simulink model "gm_HDL_pfc_gold_fi"  (R2024b)
settings: Solver=FixedStepDiscrete  StartTime=0.0  StopTime=.06  RelTol=1e-3
InitFcn:
  | fidelity_pfc_vals;
  | load('C:\Users\angro\Desktop\hil\pfc3ph\matlab\sim\sschdl\pfc_desktop\stateSpaceParameters.mat');
undefined symbols (not defined in the file or in its folder): a, b, c, fsw, t_ss, tsw
libraries: simulink x38, hdlmdlgenlib x26, hdlsllib x9, mcbcontrolslib x5, dspsrcs4 x3, slpidlib x2, spsSVPWMGenerator2LevelLib x1, spsPLL3phLib x1
(part 1 of 4)
settings Model: Creator=angro  LastModifiedBy=angro
settings OptimizationCC: BlockReduction=off  ConditionallyExecuteInputs=off  DefaultParameterBehavior=Inlined  InheritOutputTypeSmallerThanSingle=on
settings DebuggingCC: SignalRangeChecking=warning  AlgebraicLoopMsg=error  ArtificialAlgebraicLoopMsg=error  InheritedTsInSrcMsg=none  SingleTaskRateTransMsg=error  UnconnectedInputMsg=warning  UnconnectedOutputMsg=warning  UnconnectedLineMsg=warning
settings HardwareCC: ProdBitPerPointer=32  ProdBitPerSizeT=32  ProdBitPerPtrDiffT=32  ProdLargestAtomicFloat=None  ProdIntDivRoundTo=Undefined  ProdEndianess=Unspecified  ProdWordSize=32  ProdHWDeviceType=ASIC/FPGA->ASIC/FPGA  TargetBitPerPointer=64  TargetBitPerSizeT=64  TargetBitPerPtrDiffT=64  TargetLongLongMode=on  TargetIntDivRoundTo=Zero  TargetEndianess=LittleEndian  TargetWordSize=64  TargetHWDeviceType=Custom Processor->MATLAB Host Computer  ProdEqTarget=off

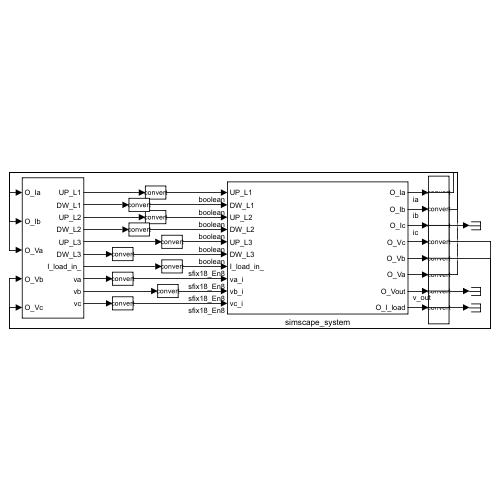
[thumbnail: Simulink's stored preview of the top-level diagram]
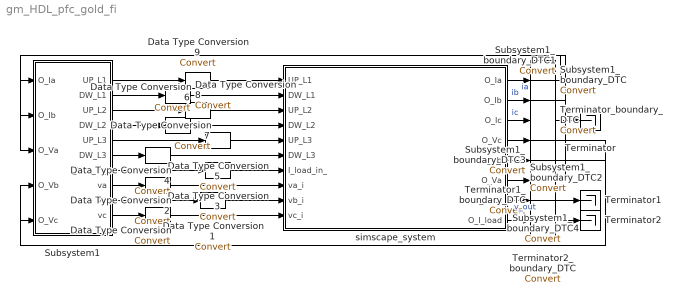
== system gm_HDL_pfc_gold_fi ==
  Data Type Conversion{,1..9} (10 alike) : DataTypeConversion  SaturateOnIntegerOverflow=off  RndMeth=Floor
  Subsystem1 : Subsystem
  Subsystem1_boundary_DTC{,1..4} (5 alike) : DataTypeConversion
  Terminator : Terminator
  Terminator1 : Terminator
  Terminator1_boundary_DTC : DataTypeConversion
  Terminator2 : Terminator
  Terminator2_boundary_DTC : DataTypeConversion
  Terminator_boundary_DTC : DataTypeConversion
  simscape_system : Subsystem
  wires:
  Terminator2_boundary_DTC/1 -> Terminator2/1
  simscape_system/8(O_I_load) -> Terminator2_boundary_DTC/1
  Terminator1_boundary_DTC/1 -> Terminator1/1
  simscape_system/7(O_Vout) -> Terminator1_boundary_DTC/1  "v_out"
  Subsystem1_boundary_DTC4/1 -> Subsystem1/3(O_Va)
  simscape_system/6(O_Va) -> Subsystem1_boundary_DTC4/1
  Subsystem1_boundary_DTC3/1 -> Subsystem1/4(O_Vb)
  simscape_system/5(O_Vb) -> Subsystem1_boundary_DTC3/1
  Subsystem1_boundary_DTC2/1 -> Subsystem1/5(O_Vc)
  simscape_system/4(O_Vc) -> Subsystem1_boundary_DTC2/1
  Terminator_boundary_DTC/1 -> Terminator/1
  simscape_system/3(O_Ic) -> Terminator_boundary_DTC/1  "ic"
  Subsystem1_boundary_DTC1/1 -> Subsystem1/2(O_Ib)
  simscape_system/2(O_Ib) -> Subsystem1_boundary_DTC1/1  "ib"
  Subsystem1_boundary_DTC/1 -> Subsystem1/1(O_Ia)
  simscape_system/1(O_Ia) -> Subsystem1_boundary_DTC/1  "ia"
  Data Type Conversion9/1 -> simscape_system/1(UP_L1)
  Data Type Conversion8/1 -> simscape_system/2(DW_L1)
  Data Type Conversion7/1 -> simscape_system/3(UP_L2)
  Data Type Conversion6/1 -> simscape_system/4(DW_L2)
  Data Type Conversion5/1 -> simscape_system/5(UP_L3)
  Data Type Conversion4/1 -> simscape_system/6(DW_L3)
  Data Type Conversion3/1 -> simscape_system/7(I_load_in_)
  Data Type Conversion2/1 -> simscape_system/8(va_i)
  Data Type Conversion1/1 -> simscape_system/9(vb_i)
  Data Type Conversion/1 -> simscape_system/10(vc_i)
  Subsystem1/10(vc) -> Data Type Conversion/1
  Subsystem1/9(vb) -> Data Type Conversion1/1
  Subsystem1/8(va) -> Data Type Conversion2/1
  Subsystem1/6(DW_L3) -> Data Type Conversion4/1
  Subsystem1/5(UP_L3) -> Data Type Conversion5/1
  Subsystem1/4(DW_L2) -> Data Type Conversion6/1
  Subsystem1/3(UP_L2) -> Data Type Conversion7/1
  Subsystem1/2(DW_L1) -> Data Type Conversion8/1
  Subsystem1/1(UP_L1) -> Data Type Conversion9/1
  Subsystem1/7(I_load_in_) -> Data Type Conversion3/1

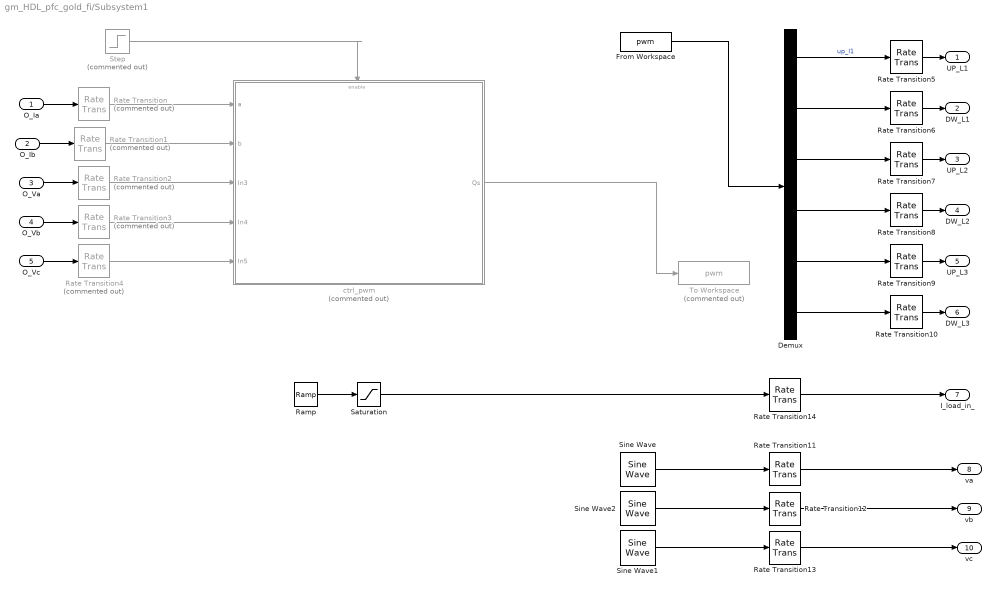
== system gm_HDL_pfc_gold_fi/Subsystem1 ==
  O_Ia : Inport
  O_Ib : Inport  Port=2
  O_Va : Inport  Port=3
  O_Vb : Inport  Port=4
  O_Vc : Inport  Port=5
  Demux : Demux  Outputs=6
  From Workspace : FromWorkspace  VariableName=pwm  SampleTime=t_ss  Interpolate=off  ZeroCross=off  OutputAfterFinalValue=Holding final value
  Ramp : simulink/Sources/Ramp  slope=1/50  start=2/50  InitialOutput=0
  Rate Transition{,1..4} (5 alike) : RateTransition  Commented=on  OutPortSampleTime=t_ss
  Rate Transition{5..10,14} (7 alike) : RateTransition  OutPortSampleTime=t_ss
  Rate Transition11 : RateTransition
  Rate Transition12 : RateTransition
  Rate Transition13 : RateTransition
  Saturation : Saturate  UpperLimit=2
  Sine Wave : dspsrcs4/Sine Wave  Amplitude=325  Frequency=50  Phase=0  SampleMode=Discrete  OutComplex=Real  CompMethod=Table lookup  TableSize=Speed  SampleTime=tsw  SamplesPerFrame=1  ResetState=Restart at time zero  OutputFrames=off  dataType=double  wordLen=16  udDataType=sfix(16)  fracBitsMode=Best precision  numFracBits=15  OutDataTypeStr=double  LastOutDataTypeStr=double
  Sine Wave1 : dspsrcs4/Sine Wave  Amplitude=325  Frequency=50  Phase=2*pi/3  SampleMode=Discrete  OutComplex=Real  CompMethod=Table lookup  TableSize=Speed  SampleTime=tsw  SamplesPerFrame=1  ResetState=Restart at time zero  OutputFrames=off  dataType=double  wordLen=16  udDataType=sfix(16)  fracBitsMode=Best precision  numFracBits=15  OutDataTypeStr=double  LastOutDataTypeStr=double
  Sine Wave2 : dspsrcs4/Sine Wave  Amplitude=325  Frequency=50  Phase=-2*pi/3  SampleMode=Discrete  OutComplex=Real  CompMethod=Table lookup  TableSize=Speed  SampleTime=tsw  SamplesPerFrame=1  ResetState=Restart at time zero  OutputFrames=off  dataType=double  wordLen=16  udDataType=sfix(16)  fracBitsMode=Best precision  numFracBits=15  OutDataTypeStr=double  LastOutDataTypeStr=double
  Step : Step  Commented=on  Time=2/50  SampleTime=0
  To Workspace : ToWorkspace  Commented=on  VariableName=pwm  SaveFormat=Timeseries  SampleTime=-1
  ctrl_pwm : Subsystem  Commented=on
  UP_L1 : Outport
  DW_L1 : Outport  Port=2
  UP_L2 : Outport  Port=3
  DW_L2 : Outport  Port=4
  UP_L3 : Outport  Port=5
  DW_L3 : Outport  Port=6
  I_load_in_ : Outport  Port=7
  va : Outport  Port=8
  vb : Outport  Port=9
  vc : Outport  Port=10
  wires:
  From Workspace/1 -> Demux/1
  Ramp/1 -> Saturation/1
  Rate Transition14/1 -> I_load_in_/1
  Step/1 -> ctrl_pwm/Enable
  Rate Transition4/1 -> ctrl_pwm/5(In5)
  Rate Transition3/1 -> ctrl_pwm/4(In4)
  Rate Transition2/1 -> ctrl_pwm/3(In3)
  Rate Transition1/1 -> ctrl_pwm/2(b)
  Rate Transition/1 -> ctrl_pwm/1(a)
  ctrl_pwm/1(Qs) -> To Workspace/1
  Rate Transition13/1 -> vc/1
  Rate Transition12/1 -> vb/1
  Rate Transition11/1 -> va/1
  Sine Wave1/1 -> Rate Transition13/1
  Sine Wave2/1 -> Rate Transition12/1
  Sine Wave/1 -> Rate Transition11/1
  Saturation/1 -> Rate Transition14/1
  Rate Transition10/1 -> DW_L3/1
  Rate Transition9/1 -> UP_L3/1
  Rate Transition8/1 -> DW_L2/1
  Rate Transition7/1 -> UP_L2/1
  Rate Transition6/1 -> DW_L1/1
  Rate Transition5/1 -> UP_L1/1
  O_Vc/1 -> Rate Transition4/1
  O_Vb/1 -> Rate Transition3/1
  O_Va/1 -> Rate Transition2/1
  O_Ib/1 -> Rate Transition1/1
  O_Ia/1 -> Rate Transition/1
  Demux/2 -> Rate Transition6/1
  Demux/3 -> Rate Transition7/1
  Demux/4 -> Rate Transition8/1
  Demux/6 -> Rate Transition10/1
  Demux/1 -> Rate Transition5/1  "up_l1"
  Demux/5 -> Rate Transition9/1

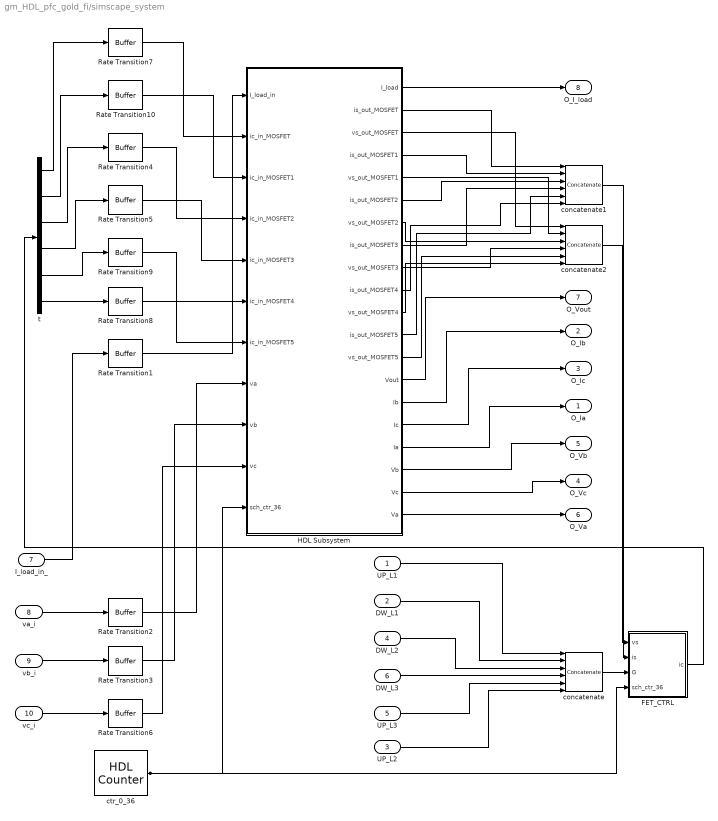
== system gm_HDL_pfc_gold_fi/simscape_system ==
  UP_L1 : Inport  OutDataTypeStr=boolean  PortDimensions=1  SampleTime=5.12820512820513e-07
  DW_L1 : Inport  Port=2  OutDataTypeStr=boolean  PortDimensions=1  SampleTime=5.12820512820513e-07
  UP_L2 : Inport  Port=3  OutDataTypeStr=boolean  PortDimensions=1  SampleTime=5.12820512820513e-07
  DW_L2 : Inport  Port=4  OutDataTypeStr=boolean  PortDimensions=1  SampleTime=5.12820512820513e-07
  UP_L3 : Inport  Port=5  OutDataTypeStr=boolean  PortDimensions=1  SampleTime=5.12820512820513e-07
  DW_L3 : Inport  Port=6  OutDataTypeStr=boolean  PortDimensions=1  SampleTime=5.12820512820513e-07
  I_load_in_ : Inport  Port=7  OutDataTypeStr=fixdt(1, 18, 8)  PortDimensions=1  SampleTime=5.12820512820513e-07
  va_i : Inport  Port=8  OutDataTypeStr=fixdt(1, 18, 8)  PortDimensions=1  SampleTime=5.12820512820513e-07  LockScale=on
  vb_i : Inport  Port=9  OutDataTypeStr=fixdt(1, 18, 8)  PortDimensions=1  SampleTime=5.12820512820513e-07  LockScale=on
  vc_i : Inport  Port=10  OutDataTypeStr=fixdt(1, 18, 8)  PortDimensions=1  SampleTime=5.12820512820513e-07  LockScale=on
  FET_CTRL : Subsystem
  HDL Subsystem : Subsystem
  Rate Transition{1..10} (10 alike) : hdlmdlgenlib/Buffer
  concatenate : Concatenate  NumInputs=6
  concatenate1 : Concatenate  NumInputs=6
  concatenate2 : Concatenate  NumInputs=6
  ctr_0_36 : hdlsllib/Sources/HDL Counter  CountType=Count limited  CountInit=double(0)  CountStep=double(1)  CountMax=double(36)  CountFromType=Initial value  CountFrom=double(0)  CountResetPort=off  CountLoadPort=off  CountEnbPort=off  CountDirPort=off  CountHitOutputPort=off  CountDataType=Unsigned  CountWordLen=6  CountFracLen=0  CountSampTime=1.38600138600139e-08
  t : Demux  Outputs=6
  O_Ia : Outport  SampleTime=5.12820512820513e-07
  O_Ib : Outport  Port=2  SampleTime=5.12820512820513e-07
  O_Ic : Outport  Port=3  SampleTime=5.12820512820513e-07
  O_Vc : Outport  Port=4  SampleTime=5.12820512820513e-07
  O_Vb : Outport  Port=5  SampleTime=5.12820512820513e-07
  O_Va : Outport  Port=6  SampleTime=5.12820512820513e-07
  O_Vout : Outport  Port=7  SampleTime=5.12820512820513e-07
  O_I_load : Outport  Port=8  SampleTime=5.12820512820513e-07
  wires:
  t/1 -> Rate Transition7/1
  t/2 -> Rate Transition10/1
  va_i/1 -> Rate Transition2/1
  concatenate/1 -> FET_CTRL/3(G)
  HDL Subsystem/12(is_out_MOSFET5) -> concatenate1/5
  t/3 -> Rate Transition4/1
  t/4 -> Rate Transition5/1
  t/5 -> Rate Transition9/1
  t/6 -> Rate Transition8/1
  I_load_in_/1 -> Rate Transition1/1
  UP_L1/1 -> concatenate/1
  vb_i/1 -> Rate Transition3/1
  DW_L1/1 -> concatenate/2
  Rate Transition2/1 -> HDL Subsystem/8(va)
  vc_i/1 -> Rate Transition6/1
  Rate Transition10/1 -> HDL Subsystem/3(ic_in_MOSFET1)
  Rate Transition7/1 -> HDL Subsystem/2(ic_in_MOSFET)
  HDL Subsystem/10(is_out_MOSFET4) -> concatenate1/6
  Rate Transition4/1 -> HDL Subsystem/4(ic_in_MOSFET2)
  Rate Transition5/1 -> HDL Subsystem/5(ic_in_MOSFET3)
  Rate Transition9/1 -> HDL Subsystem/7(ic_in_MOSFET5)
  Rate Transition8/1 -> HDL Subsystem/6(ic_in_MOSFET4)
  Rate Transition3/1 -> HDL Subsystem/9(vb)
  Rate Transition1/1 -> HDL Subsystem/1(I_load_in)
  HDL Subsystem/13(vs_out_MOSFET5) -> concatenate2/5
  Rate Transition6/1 -> HDL Subsystem/10(vc)
  concatenate2/1 -> FET_CTRL/1(vs)
  HDL Subsystem/17(Ia) -> O_Ia/1
  ctr_0_36/1 -> HDL Subsystem/11(sch_ctr_36), FET_CTRL/4(sch_ctr_36)
  HDL Subsystem/1(I_load) -> O_I_load/1
  HDL Subsystem/2(is_out_MOSFET) -> concatenate1/1
  HDL Subsystem/3(vs_out_MOSFET) -> concatenate2/1
  HDL Subsystem/4(is_out_MOSFET1) -> concatenate1/2
  HDL Subsystem/5(vs_out_MOSFET1) -> concatenate2/2
  UP_L3/1 -> concatenate/5
  HDL Subsystem/6(is_out_MOSFET2) -> concatenate1/3
  HDL Subsystem/7(vs_out_MOSFET2) -> concatenate2/3
  HDL Subsystem/8(is_out_MOSFET3) -> concatenate1/4
  concatenate1/1 -> FET_CTRL/2(is)
  HDL Subsystem/9(vs_out_MOSFET3) -> concatenate2/4
  UP_L2/1 -> concatenate/6
  HDL Subsystem/11(vs_out_MOSFET4) -> concatenate2/6
  HDL Subsystem/14(Vout) -> O_Vout/1
  HDL Subsystem/15(Ib) -> O_Ib/1
  HDL Subsystem/16(Ic) -> O_Ic/1
  HDL Subsystem/18(Vb) -> O_Vb/1
  DW_L3/1 -> concatenate/4
  HDL Subsystem/19(Vc) -> O_Vc/1
  HDL Subsystem/20(Va) -> O_Va/1
  DW_L2/1 -> concatenate/3
  FET_CTRL/1(ic) -> t/1

== system gm_HDL_pfc_gold_fi/Subsystem1/ctrl_pwm ==
  a : Inport
  b : Inport  Port=2
  In3 : Inport  Port=3
  In4 : Inport  Port=4
  In5 : Inport  Port=5
  Enable : EnablePort
  PI_CTRL : Subsystem
  SVPWM : Subsystem
  transforms : Subsystem
  Qs : Outport
  wires:
  In4/1 -> transforms/4(In4)
  In3/1 -> transforms/3(In3)
  b/1 -> transforms/2(b)
  PI_CTRL/2(Vq_inductor) -> SVPWM/3(Vq_inductor)
  SVPWM/1(P) -> Qs/1  "Qs"
  transforms/2(iq) -> PI_CTRL/2(iq)
  In5/1 -> transforms/5(In5)
  a/1 -> transforms/1(a)
  PI_CTRL/1(Vd_inductor) -> SVPWM/1(Vd_inductor)
  transforms/3(angle) -> SVPWM/2(angle)
  transforms/1(id) -> PI_CTRL/1(id)

== system gm_HDL_pfc_gold_fi/simscape_system/FET_CTRL ==
  vs : Inport  OutDataTypeStr=fixdt(1, 18, 6)  PortDimensions=[6]  SampleTime=1.38600138600139e-08
  is : Inport  Port=2  OutDataTypeStr=fixdt(1, 18, 6)  PortDimensions=[6]  SampleTime=1.38600138600139e-08
  G : Inport  Port=3  OutDataTypeStr=boolean  PortDimensions=[6]  SampleTime=5.12820512820513e-07
  sch_ctr_36 : Inport  Port=4  OutDataTypeStr=fixdt(0, 6, 0)  SampleTime=1.38600138600139e-08
  Discrete-Time Integrator_reg : RateTransition  InitialCondition=double(0)  OutPortSampleTimeOpt=Multiple of input port sample time  OutPortSampleTimeMultiple=37
  Discrete-Time Integrator_reg_absorbed : Delay  DelayLength=0
  crp_temp_streamed : Subsystem
  in0_repeat : RateTransition  Integrity=off  Deterministic=off  OutPortSampleTimeOpt=Multiple of input port sample time  OutPortSampleTimeMultiple=1/37
  in3_repeat : RateTransition  Integrity=off  Deterministic=off  OutPortSampleTimeOpt=Multiple of input port sample time  OutPortSampleTimeMultiple=1/37
  ic : Outport  SampleTime=1.38600138600139e-08
  wires:
  G/1 -> in3_repeat/1
  vs/1 -> crp_temp_streamed/3(in2)
  in3_repeat/1 -> crp_temp_streamed/2(in1)
  crp_temp_streamed/1(out0) -> Discrete-Time Integrator_reg/1
  is/1 -> crp_temp_streamed/4(in3)
  sch_ctr_36/1 -> crp_temp_streamed/5(enb_counter)
  in0_repeat/1 -> crp_temp_streamed/1(in0)
  crp_temp_streamed/2(out1) -> ic/1
  Discrete-Time Integrator_reg/1 -> Discrete-Time Integrator_reg_absorbed/1
  Discrete-Time Integrator_reg_absorbed/1 -> in0_repeat/1

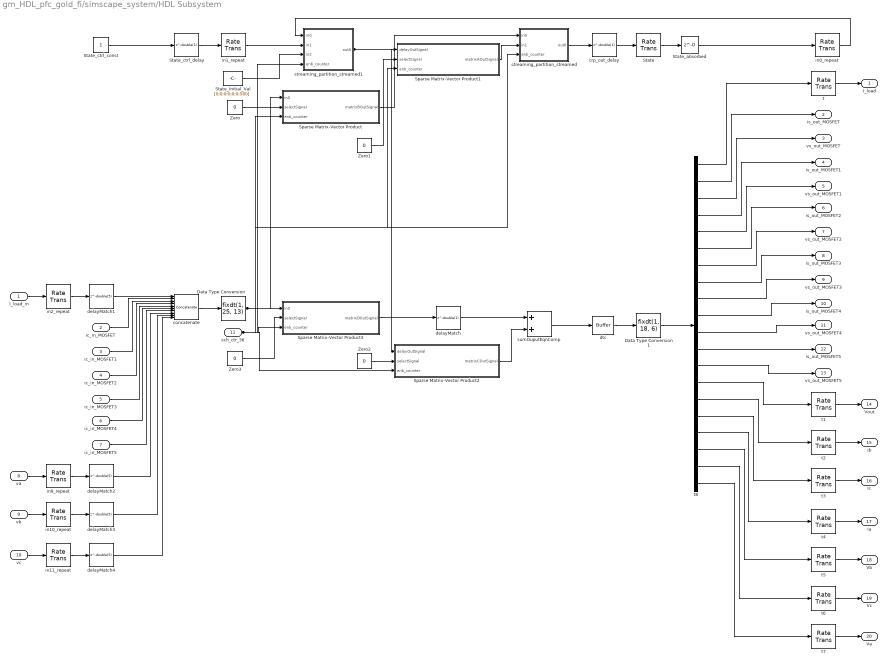
== system gm_HDL_pfc_gold_fi/simscape_system/HDL Subsystem ==
  I_load_in : Inport  OutDataTypeStr=fixdt(1, 18, 8)  PortDimensions=1  SampleTime=5.12820512820513e-07
  ic_in_MOSFET : Inport  Port=2  OutDataTypeStr=fixdt(1, 18, 8)  PortDimensions=1  SampleTime=1.38600138600139e-08
  ic_in_MOSFET1 : Inport  Port=3  OutDataTypeStr=fixdt(1, 18, 8)  PortDimensions=1  SampleTime=1.38600138600139e-08
  ic_in_MOSFET2 : Inport  Port=4  OutDataTypeStr=fixdt(1, 18, 8)  PortDimensions=1  SampleTime=1.38600138600139e-08
  ic_in_MOSFET3 : Inport  Port=5  OutDataTypeStr=fixdt(1, 18, 8)  PortDimensions=1  SampleTime=1.38600138600139e-08
  ic_in_MOSFET4 : Inport  Port=6  OutDataTypeStr=fixdt(1, 18, 8)  PortDimensions=1  SampleTime=1.38600138600139e-08
  ic_in_MOSFET5 : Inport  Port=7  OutDataTypeStr=fixdt(1, 18, 8)  PortDimensions=1  SampleTime=1.38600138600139e-08
  va : Inport  Port=8  OutDataTypeStr=fixdt(1, 18, 8)  PortDimensions=1  SampleTime=5.12820512820513e-07
  vb : Inport  Port=9  OutDataTypeStr=fixdt(1, 18, 8)  PortDimensions=1  SampleTime=5.12820512820513e-07
  vc : Inport  Port=10  OutDataTypeStr=fixdt(1, 18, 8)  PortDimensions=1  SampleTime=5.12820512820513e-07
  sch_ctr_36 : Inport  Port=11  OutDataTypeStr=fixdt(0, 6, 0)  SampleTime=1.38600138600139e-08
  Data Type Conversion : DataTypeConversion  OutDataTypeStr=fixdt(1, 25, 13)  SampleTime=1.38600138600139e-08  SaturateOnIntegerOverflow=off  RndMeth=Floor
  Data Type Conversion1 : DataTypeConversion  OutDataTypeStr=fixdt(1, 18, 6)  SampleTime=1.38600138600139e-08  SaturateOnIntegerOverflow=off  RndMeth=Floor
  Sparse Matrix-Vector Product : Subsystem
  Sparse Matrix-Vector Product1 : Subsystem
  Sparse Matrix-Vector Product2 : Subsystem
  Sparse Matrix-Vector Product3 : Subsystem
  State : RateTransition  InitialCondition=double(0)  OutPortSampleTimeOpt=Multiple of input port sample time  OutPortSampleTimeMultiple=37
  State_Initial_Val : Constant  Value=[0;0;0;0;0;0;580]  OutDataTypeStr=fixdt(1, 25, 13)  SampleTime=1.38600138600139e-08
  State_absorbed : Delay  DelayLength=0
  State_ctrl_const : Constant  OutDataTypeStr=boolean  SampleTime=5.12820512820513e-07
  State_ctrl_delay : Delay  DelayLength=double(1)  InitialCondition=0  SampleTime=5.12820512820513e-07
  Zero{,1..3} (4 alike) : Constant  Value=0  OutDataTypeStr=boolean  SampleTime=1.38600138600139e-08
  concatenate : Concatenate  NumInputs=10
  crp_out_delay : Delay  DelayLength=double(1)  InitialCondition=0  SampleTime=1.38600138600139e-08
  delayMatch : Delay  DelayLength=double(1)  InitialCondition=0  SampleTime=1.38600138600139e-08
  delayMatch{1..4} (4 alike) : Delay  DelayLength=double(5)  InitialCondition=0  SampleTime=1.38600138600139e-08
  dtc : hdlmdlgenlib/Buffer
  in0_repeat : RateTransition  Integrity=off  Deterministic=off  OutPortSampleTimeOpt=Multiple of input port sample time  OutPortSampleTimeMultiple=1/37
  in10_repeat : RateTransition  Integrity=off  Deterministic=off  OutPortSampleTimeOpt=Multiple of input port sample time  OutPortSampleTimeMultiple=1/37
  in11_repeat : RateTransition  Integrity=off  Deterministic=off  OutPortSampleTimeOpt=Multiple of input port sample time  OutPortSampleTimeMultiple=1/37
  in1_repeat : RateTransition  Integrity=off  Deterministic=off  OutPortSampleTimeOpt=Multiple of input port sample time  OutPortSampleTimeMultiple=1/37
  in2_repeat : RateTransition  Integrity=off  Deterministic=off  OutPortSampleTimeOpt=Multiple of input port sample time  OutPortSampleTimeMultiple=1/37
  in9_repeat : RateTransition  Integrity=off  Deterministic=off  OutPortSampleTimeOpt=Multiple of input port sample time  OutPortSampleTimeMultiple=1/37
  streaming_partition_streamed : Subsystem
  streaming_partition_streamed1 : Subsystem
  sumOuputEqnComp : Sum  OutDataTypeStr=fixdt(1, 25, 13)  SampleTime=1.38600138600139e-08
  t{,1..7} (8 alike) : RateTransition  InitialCondition=double(0)  OutPortSampleTimeOpt=Multiple of input port sample time  OutPortSampleTimeMultiple=37
  t8 : Demux  Outputs=20
  I_load : Outport  SampleTime=5.12820512820513e-07
  is_out_MOSFET : Outport  Port=2  SampleTime=1.38600138600139e-08
  vs_out_MOSFET : Outport  Port=3  SampleTime=1.38600138600139e-08
  is_out_MOSFET1 : Outport  Port=4  SampleTime=1.38600138600139e-08
  vs_out_MOSFET1 : Outport  Port=5  SampleTime=1.38600138600139e-08
  is_out_MOSFET2 : Outport  Port=6  SampleTime=1.38600138600139e-08
  vs_out_MOSFET2 : Outport  Port=7  SampleTime=1.38600138600139e-08
  is_out_MOSFET3 : Outport  Port=8  SampleTime=1.38600138600139e-08
  vs_out_MOSFET3 : Outport  Port=9  SampleTime=1.38600138600139e-08
  is_out_MOSFET4 : Outport  Port=10  SampleTime=1.38600138600139e-08
  vs_out_MOSFET4 : Outport  Port=11  SampleTime=1.38600138600139e-08
  is_out_MOSFET5 : Outport  Port=12  SampleTime=1.38600138600139e-08
  vs_out_MOSFET5 : Outport  Port=13  SampleTime=1.38600138600139e-08
  Vout : Outport  Port=14  SampleTime=5.12820512820513e-07
  Ib : Outport  Port=15  SampleTime=5.12820512820513e-07
  Ic : Outport  Port=16  SampleTime=5.12820512820513e-07
  Ia : Outport  Port=17  SampleTime=5.12820512820513e-07
  Vb : Outport  Port=18  SampleTime=5.12820512820513e-07
  Vc : Outport  Port=19  SampleTime=5.12820512820513e-07
  Va : Outport  Port=20  SampleTime=5.12820512820513e-07
  wires:
  crp_out_delay/1 -> State/1
  I_load_in/1 -> in2_repeat/1
  in11_repeat/1 -> delayMatch4/1
  Sparse Matrix-Vector Product/1(matrixBOutSignal) -> streaming_partition_streamed/1(in0)
  va/1 -> in9_repeat/1
  in9_repeat/1 -> delayMatch2/1
  Sparse Matrix-Vector Product1/1(matrixAOutSignal) -> streaming_partition_streamed/2(in1)
  Zero/1 -> Sparse Matrix-Vector Product/2(selectSignal)
  vb/1 -> in10_repeat/1
  t5/1 -> Vb/1
  ic_in_MOSFET/1 -> concatenate/2
  vc/1 -> in11_repeat/1
  t8/16 -> t3/1
  t8/15 -> t2/1
  in2_repeat/1 -> delayMatch1/1
  in10_repeat/1 -> delayMatch3/1
  ic_in_MOSFET3/1 -> concatenate/5
  State_ctrl_const/1 -> State_ctrl_delay/1
  delayMatch1/1 -> concatenate/1
  ic_in_MOSFET4/1 -> concatenate/6
  ic_in_MOSFET1/1 -> concatenate/3
  ic_in_MOSFET2/1 -> concatenate/4
  Data Type Conversion1/1 -> t8/1
  ic_in_MOSFET5/1 -> concatenate/7
  t8/10 -> is_out_MOSFET4/1
  t8/9 -> vs_out_MOSFET3/1
  delayMatch2/1 -> concatenate/8
  t8/20 -> t7/1
  delayMatch3/1 -> concatenate/9
  t8/19 -> t6/1
  delayMatch4/1 -> concatenate/10
  State_ctrl_delay/1 -> in1_repeat/1
  concatenate/1 -> Data Type Conversion/1
  in1_repeat/1 -> streaming_partition_streamed1/2(in1)
  State_Initial_Val/1 -> streaming_partition_streamed1/3(in2)
  Data Type Conversion/1 -> Sparse Matrix-Vector Product/1(in0), Sparse Matrix-Vector Product3/1(in0)
  sch_ctr_36/1 -> Sparse Matrix-Vector Product2/3(enb_counter), Sparse Matrix-Vector Product3/3(enb_counter), streaming_partition_streamed1/4(enb_counter), Sparse Matrix-Vector Product/3(enb_counter), Sparse Matrix-Vector Product1/3(enb_counter), streaming_partition_streamed/3(enb_counter)
  Zero3/1 -> Sparse Matrix-Vector Product3/2(selectSignal)
  streaming_partition_streamed1/1(out0) -> Sparse Matrix-Vector Product2/1(delayOutSignal), Sparse Matrix-Vector Product1/1(delayOutSignal)
  Zero1/1 -> Sparse Matrix-Vector Product1/2(selectSignal)
  t8/18 -> t5/1
  Sparse Matrix-Vector Product3/1(matrixDOutSignal) -> delayMatch/1
  t8/17 -> t4/1
  Sparse Matrix-Vector Product2/1(matrixCOutSignal) -> sumOuputEqnComp/2
  Zero2/1 -> Sparse Matrix-Vector Product2/2(selectSignal)
  delayMatch/1 -> sumOuputEqnComp/1
  t8/4 -> is_out_MOSFET1/1
  streaming_partition_streamed/1(out0) -> crp_out_delay/1
  sumOuputEqnComp/1 -> dtc/1
  dtc/1 -> Data Type Conversion1/1
  State/1 -> State_absorbed/1
  State_absorbed/1 -> in0_repeat/1
  t8/2 -> is_out_MOSFET/1
  t8/1 -> t/1
  t8/3 -> vs_out_MOSFET/1
  t8/6 -> is_out_MOSFET2/1
  t8/5 -> vs_out_MOSFET1/1
  t8/8 -> is_out_MOSFET3/1
  t8/7 -> vs_out_MOSFET2/1
  in0_repeat/1 -> streaming_partition_streamed1/1(in0)
  t8/12 -> is_out_MOSFET5/1
  t8/11 -> vs_out_MOSFET4/1
  t8/14 -> t1/1
  t8/13 -> vs_out_MOSFET5/1
  t/1 -> I_load/1
  t1/1 -> Vout/1
  t2/1 -> Ib/1
  t3/1 -> Ic/1
  t4/1 -> Ia/1
  t6/1 -> Vc/1
  t7/1 -> Va/1

== system gm_HDL_pfc_gold_fi/Subsystem1/ctrl_pwm/PI_CTRL ==
  id : Inport
  iq : Inport  Port=2
  Add3 : Sum  Inputs=+-
  Add4 : Sum  Inputs=+-
  Constant : Constant  Value=0  SampleTime=t_ss
  Constant1 : Constant  Value=-6  SampleTime=t_ss
  Vd_ctrl : slpidlib/PID Controller  Controller=PI  Form=Parallel  TimeDomain=Discrete-time  UseExternalTs=off  SampleTime=t_ss  IntegratorMethod=Backward Euler  FilterMethod=Forward Euler  ControllerParametersSource=internal  P=-1.8  I=-.15  UseKiTs=off  D=0  UseExternalDerivativeSource=off  N=100  UseFilter=on  TunerSelectOption=Transfer Function Based (PID Tuner App)  InitialConditionSource=internal  InitialConditionForIntegrator=0  InitialConditionForFilter=0  DifferentiatorICPrevScaledInput=0  ExternalReset=none  TrackingMode=off  Kt=1  LimitOutput=off  SatLimitsSource=internal  UpperSaturationLimit=5e2  LowerSaturationLimit=-5e2  LinearizeAsGain=on  AntiWindupMode=clamping  Kb=1  LimitIntegrator=off  UpperIntegratorSaturationLimit=inf  LowerIntegratorSaturationLimit=-inf  POutMin=[]  POutMax=[]  IOutMin=[]  IOutMax=[]  DOutMin=[]  DOutMax=[]  NOutMin=[]  NOutMax=[]  SumOutMin=[]  SumOutMax=[]  SaturationOutMin=[]  SaturationOutMax=[]  PParamMin=[]  PParamMax=[]  IParamMin=[]  IParamMax=[]  DParamMin=[]  DParamMax=[]  NParamMin=[]  NParamMax=[]  KbParamMin=[]  KbParamMax=[]  KtParamMin=[]  KtParamMax=[]  KbOutMin=[]  KbOutMax=[]  KtOutMin=[]  KtOutMax=[]  IntegratorOutMin=[]  IntegratorOutMax=[]  FilterOutMin=[]  FilterOutMax=[]  SumI1OutMin=[]  SumI1OutMax=[]  SumI2OutMin=[]  SumI2OutMax=[]  SumI3OutMin=[]  SumI3OutMax=[]  SumI4OutMin=[]  SumI4OutMax=[]  SumDOutMin=[]  SumDOutMax=[]  DifferentiatorOutMin=[]  DifferentiatorOutMax=[]  FilterDiffOutCoefMin=[]  FilterDiffOutCoefMax=[]  ReciprocalOutMin=[]  ReciprocalOutMax=[]  SumDenOutMin=[]  SumDenOutMax=[]  SumNumOutMin=[]  SumNumOutMax=[]  DivideOutMin=[]  DivideOutMax=[]  UdiffTsProdOutMin=[]  UdiffTsProdOutMax=[]  NTsProdOutMin=[]  NTsProdOutMax=[]  UintegralTsProdOutMin=[]  UintegralTsProdOutMax=[]  UngainTsProdOutMin=[]  UngainTsProdOutMax=[]  ClampingZeroOutDataTypeStr=Inherit: Inherit via back propagation  ClampingZeroOutMin=[]  ClampingZeroOutMax=[]  FilterDenConstantOutDataTypeStr=Inherit: Inherit via back propagation  FilterDenConstantOutMin=[]  FilterDenConstantOutMax=[]  PCopyOutDataTypeStr=Inherit: Inherit via back propagation  PCopyOutMin=[]  PCopyOutMax=[]  NCopyOutDataTypeStr=Inherit: Inherit via back propagation  NCopyOutMin=[]  NCopyOutMax=[]  IntegratorContinuousStateAttributes=''  IntegratorStateMustResolveToSignalObject=off  IntegratorRTWStateStorageClass=Auto  FilterContinuousStateAttributes=''  FilterStateMustResolveToSignalObject=off  FilterRTWStateStorageClass=Auto  ParallelPVariant=InternalParameters  IdealPVariant=Disabled  IVariant=InternalParameters  DVariant=Disabled  IntegratorVariant=Discrete  SatVariant=Disabled  AWVariant=Passthrough  PCopyVariant=Disabled  TRVariant=Disabled  FdbkBlocksVariant=Forward  IdealPFdbkVariant=Disabled  SatFdbkVariant=Disabled  DerivativeFilterVariant=Disabled  NVariant=Disabled  NCopyVariant=Disabled_SignalSpec  FilterICVariant=Disabled  IntegratorICVariant=InternalICs  ExternalResetVariant=Disabled  TRSumVariant=Passthrough  SumFdbkVariant=Disabled  SumVariant=Sum_PI  TsampFilterVariant=InternalTs  TsampNgainVariant=Passthrough  TsampIntegralVariant=Disabled_SignalSpec  ExternalSaturationOutDataTypeStr=Inherit: Same as second input  DerivativeSourceVariant=Disabled  PreIntVariant=InternalPreInt
  Vq_ctrl : slpidlib/PID Controller  Controller=PI  Form=Parallel  TimeDomain=Discrete-time  UseExternalTs=off  SampleTime=t_ss  IntegratorMethod=Backward Euler  FilterMethod=Forward Euler  ControllerParametersSource=internal  P=-2  I=-.2  UseKiTs=off  D=0  UseExternalDerivativeSource=off  N=100  UseFilter=on  TunerSelectOption=Transfer Function Based (PID Tuner App)  InitialConditionSource=internal  InitialConditionForIntegrator=0  InitialConditionForFilter=0  DifferentiatorICPrevScaledInput=0  ExternalReset=none  TrackingMode=off  Kt=1  LimitOutput=off  SatLimitsSource=internal  UpperSaturationLimit=5e2  LowerSaturationLimit=-5e2  LinearizeAsGain=on  AntiWindupMode=clamping  Kb=1  LimitIntegrator=off  UpperIntegratorSaturationLimit=inf  LowerIntegratorSaturationLimit=-inf  POutMin=[]  POutMax=[]  IOutMin=[]  IOutMax=[]  DOutMin=[]  DOutMax=[]  NOutMin=[]  NOutMax=[]  SumOutMin=[]  SumOutMax=[]  SaturationOutMin=[]  SaturationOutMax=[]  PParamMin=[]  PParamMax=[]  IParamMin=[]  IParamMax=[]  DParamMin=[]  DParamMax=[]  NParamMin=[]  NParamMax=[]  KbParamMin=[]  KbParamMax=[]  KtParamMin=[]  KtParamMax=[]  KbOutMin=[]  KbOutMax=[]  KtOutMin=[]  KtOutMax=[]  IntegratorOutMin=[]  IntegratorOutMax=[]  FilterOutMin=[]  FilterOutMax=[]  SumI1OutMin=[]  SumI1OutMax=[]  SumI2OutMin=[]  SumI2OutMax=[]  SumI3OutMin=[]  SumI3OutMax=[]  SumI4OutMin=[]  SumI4OutMax=[]  SumDOutMin=[]  SumDOutMax=[]  DifferentiatorOutMin=[]  DifferentiatorOutMax=[]  FilterDiffOutCoefMin=[]  FilterDiffOutCoefMax=[]  ReciprocalOutMin=[]  ReciprocalOutMax=[]  SumDenOutMin=[]  SumDenOutMax=[]  SumNumOutMin=[]  SumNumOutMax=[]  DivideOutMin=[]  DivideOutMax=[]  UdiffTsProdOutMin=[]  UdiffTsProdOutMax=[]  NTsProdOutMin=[]  NTsProdOutMax=[]  UintegralTsProdOutMin=[]  UintegralTsProdOutMax=[]  UngainTsProdOutMin=[]  UngainTsProdOutMax=[]  ClampingZeroOutDataTypeStr=Inherit: Inherit via back propagation  ClampingZeroOutMin=[]  ClampingZeroOutMax=[]  FilterDenConstantOutDataTypeStr=Inherit: Inherit via back propagation  FilterDenConstantOutMin=[]  FilterDenConstantOutMax=[]  PCopyOutDataTypeStr=Inherit: Inherit via back propagation  PCopyOutMin=[]  PCopyOutMax=[]  NCopyOutDataTypeStr=Inherit: Inherit via back propagation  NCopyOutMin=[]  NCopyOutMax=[]  IntegratorContinuousStateAttributes=''  IntegratorStateMustResolveToSignalObject=off  IntegratorRTWStateStorageClass=Auto  FilterContinuousStateAttributes=''  FilterStateMustResolveToSignalObject=off  FilterRTWStateStorageClass=Auto  ParallelPVariant=InternalParameters  IdealPVariant=Disabled  IVariant=InternalParameters  DVariant=Disabled  IntegratorVariant=Discrete  SatVariant=Disabled  AWVariant=Passthrough  PCopyVariant=Disabled  TRVariant=Disabled  FdbkBlocksVariant=Forward  IdealPFdbkVariant=Disabled  SatFdbkVariant=Disabled  DerivativeFilterVariant=Disabled  NVariant=Disabled  NCopyVariant=Disabled_SignalSpec  FilterICVariant=Disabled  IntegratorICVariant=InternalICs  ExternalResetVariant=Disabled  TRSumVariant=Passthrough  SumFdbkVariant=Disabled  SumVariant=Sum_PI  TsampFilterVariant=InternalTs  TsampNgainVariant=Passthrough  TsampIntegralVariant=Disabled_SignalSpec  ExternalSaturationOutDataTypeStr=Inherit: Same as second input  DerivativeSourceVariant=Disabled  PreIntVariant=InternalPreInt
  Vd_inductor : Outport
  Vq_inductor : Outport  Port=2
  wires:
  Constant1/1 -> Add4/1
  Vq_ctrl/1 -> Vq_inductor/1
  Vd_ctrl/1 -> Vd_inductor/1
  Add4/1 -> Vq_ctrl/1  "error_iq"
  iq/1 -> Add4/2
  Constant/1 -> Add3/1
  id/1 -> Add3/2
  Add3/1 -> Vd_ctrl/1  "error_id"

== system gm_HDL_pfc_gold_fi/Subsystem1/ctrl_pwm/SVPWM ==
  Vd_inductor : Inport
  angle : Inport  Port=2
  Vq_inductor : Inport  Port=3
  Cos : Trigonometry  Operator=cos
  Inverse Park Transform : mcbcontrolslib/Inverse Park Transform  PhaseInput=Two inputs  AxisAlignment=D-axis  ThetaInput=Sine and Cosine electrical position  AngleInput=Per-unit  N_points=1024
  SVPWM Generator (2-Level) : spsSVPWMGenerator2LevelLib/SVPWM Generator (2-Level)  InputType=alpha-beta components  SwitchingPattern=Pattern #1  Fc=fsw*1e3  ParUref=[0.8 -30 50]  Ts=t_ss
  Sin : Trigonometry
  P : Outport
  wires:
  SVPWM Generator (2-Level)/1 -> P/1
  angle/1 -> Sin/1, Cos/1
  Inverse Park Transform/1 -> SVPWM Generator (2-Level)/1  "Valp_indc"
  Cos/1 -> Inverse Park Transform/4
  Sin/1 -> Inverse Park Transform/3
  Inverse Park Transform/2 -> SVPWM Generator (2-Level)/2  "Vbet_indc"
  Vq_inductor/1 -> Inverse Park Transform/2
  Vd_inductor/1 -> Inverse Park Transform/1

== system gm_HDL_pfc_gold_fi/Subsystem1/ctrl_pwm/transforms ==
  a : Inport
  b : Inport  Port=2
  In3 : Inport  Port=3
  In4 : Inport  Port=4
  In5 : Inport  Port=5
  Claro-Parl Transform : Subsystem  Commented=on
  Claro-Parl Transform1 : Subsystem
  Delay : Delay  DelayLength=1
  Delay1 : Delay  DelayLength=1
  Mux : Mux  Inputs=3
  PLL (3ph) : spsPLL3phLib/PLL (3ph)  Fmin=50  Par_Init=[0, 50]  ParK=[180,3200,1]  TcD=1e-4  MaxRateChangeFreq=12  FilterCutOffFreq=25  Ts=t_ss  AGC=on
  Terminator : Terminator
  id : Outport
  iq : Outport  Port=2
  angle : Outport  Port=3
  wires:
  Claro-Parl Transform1/2(q) -> iq/1  "iq"
  Claro-Parl Transform1/1(d) -> id/1  "id"
  Claro-Parl Transform/2(q) -> ?  "vq"
  Claro-Parl Transform/1(d) -> ?  "vd"
  Delay1/1 -> Claro-Parl Transform1/2(b)
  Delay/1 -> Claro-Parl Transform1/1(a)
  a/1 -> Delay/1
  In4/1 -> Mux/2, Claro-Parl Transform/2(b)
  b/1 -> Delay1/1
  In5/1 -> Mux/3
  In3/1 -> Claro-Parl Transform/1(a), Mux/1
  PLL (3ph)/1 -> Terminator/1
  PLL (3ph)/2 -> Claro-Parl Transform/3(wt), Claro-Parl Transform1/3(wt), angle/1  "angle"
  Mux/1 -> PLL (3ph)/1

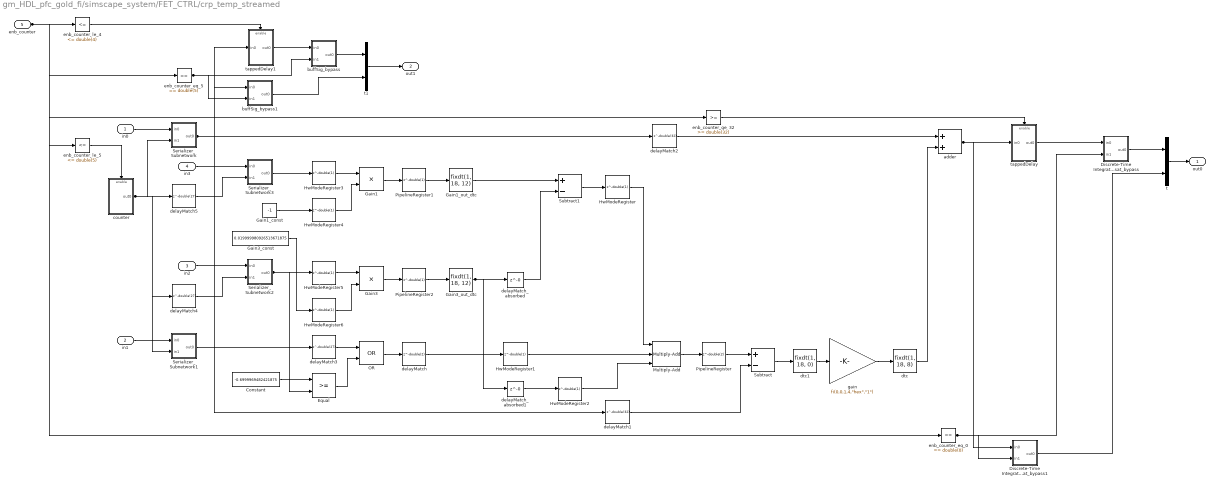
== system gm_HDL_pfc_gold_fi/simscape_system/FET_CTRL/crp_temp_streamed ==
  in0 : Inport  OutDataTypeStr=fixdt(1, 18, 8)  PortDimensions=[6]  SampleTime=1.38600138600139e-08
  in1 : Inport  Port=2  OutDataTypeStr=boolean  PortDimensions=[6]  SampleTime=1.38600138600139e-08
  in2 : Inport  Port=3  OutDataTypeStr=fixdt(1, 18, 6)  PortDimensions=[6]  SampleTime=1.38600138600139e-08
  in3 : Inport  Port=4  OutDataTypeStr=fixdt(1, 18, 6)  PortDimensions=[6]  SampleTime=1.38600138600139e-08
  enb_counter : Inport  Port=5  OutDataTypeStr=fixdt(0, 6, 0)  SampleTime=1.38600138600139e-08
  Constant : Constant  Value=-0.6999969482421875  OutDataTypeStr=fixdt(1, 18, 17)  SampleTime=1.38600138600139e-08
  Discrete-Time Integrator_u_sat_bypass : Subsystem
  Discrete-Time Integrator_u_sat_bypass1 : Subsystem
  Equal : RelationalOperator  OutDataTypeStr=boolean  SampleTime=1.38600138600139e-08  InputSameDT=off
  Gain1 : Product  Inputs=**  OutDataTypeStr=fixdt(1, 36, 23)  SampleTime=1.38600138600139e-08
  Gain1_const : Constant  Value=-1  OutDataTypeStr=fixdt(1, 18, 17)  SampleTime=1.38600138600139e-08
  Gain1_out_dtc : DataTypeConversion  OutDataTypeStr=fixdt(1, 18, 12)  SampleTime=1.38600138600139e-08  SaturateOnIntegerOverflow=off  RndMeth=Floor
  Gain3 : Product  Inputs=**  OutDataTypeStr=fixdt(1, 36, 28)  SampleTime=1.38600138600139e-08
  Gain3_const : Constant  Value=0.019999980926513671875  OutDataTypeStr=fixdt(1, 18, 22)  SampleTime=1.38600138600139e-08
  Gain3_out_dtc : DataTypeConversion  OutDataTypeStr=fixdt(1, 18, 12)  SampleTime=1.38600138600139e-08  SaturateOnIntegerOverflow=off  RndMeth=Floor
  HwModeRegister{,1..6} (7 alike) : Delay  DelayLength=double(1)  InitialCondition=0  SampleTime=1.38600138600139e-08
  Multiply-Add : hdlsllib/HDL Operations/Multiply-Add  Function=c+(a.*b)  datatype=fixdt(1, 18, 12)  DoSatur=off  FMA=off
  OR : Logic  Operator=OR  AllPortsSameDT=off  OutDataTypeStr=boolean  SampleTime=1.38600138600139e-08
  PipelineRegister : Delay  DelayLength=double(2)  InitialCondition=0  SampleTime=1.38600138600139e-08
  PipelineRegister1 : Delay  DelayLength=double(1)  InitialCondition=0  SampleTime=1.38600138600139e-08
  PipelineRegister2 : Delay  DelayLength=double(1)  InitialCondition=0  SampleTime=1.38600138600139e-08
  Serializer_Subnetwork : Subsystem
  Serializer_Subnetwork1 : Subsystem
  Serializer_Subnetwork2 : Subsystem
  Serializer_Subnetwork3 : Subsystem
  Subtract : Sum  Inputs=+-  OutDataTypeStr=fixdt(1, 18, 12)  AccumDataTypeStr=fixdt(1, 23, 12)  SampleTime=1.38600138600139e-08
  Subtract1 : Sum  Inputs=+-  OutDataTypeStr=fixdt(1, 18, 11)  AccumDataTypeStr=fixdt(1, 19, 12)  SampleTime=1.38600138600139e-08
  adder : Sum  OutDataTypeStr=fixdt(1, 18, 8)  AccumDataTypeStr=fixdt(1, 18, 8)  SampleTime=1.38600138600139e-08
  buffSig_bypass : Subsystem
  buffSig_bypass1 : Subsystem
  counter : Subsystem
  delayMatch : Delay  DelayLength=double(2)  InitialCondition=0  SampleTime=1.38600138600139e-08
  delayMatch1 : Delay  DelayLength=double(32)  InitialCondition=0  SampleTime=1.38600138600139e-08
  delayMatch2 : Delay  DelayLength=double(32)  InitialCondition=0  SampleTime=1.38600138600139e-08
  delayMatch3 : Delay  DelayLength=double(27)  InitialCondition=0  SampleTime=1.38600138600139e-08
  delayMatch4 : Delay  DelayLength=double(27)  InitialCondition=0  SampleTime=1.38600138600139e-08
  delayMatch5 : Delay  DelayLength=double(27)  InitialCondition=0  SampleTime=1.38600138600139e-08
  delayMatch_absorbed : Delay  DelayLength=0
  delayMatch_absorbed1 : Delay  DelayLength=0
  dtc : DataTypeConversion  OutDataTypeStr=fixdt(1, 18, 8)  ConvertRealWorld=Stored Integer (SI)  SampleTime=1.38600138600139e-08  SaturateOnIntegerOverflow=off  RndMeth=Floor
  dtc1 : DataTypeConversion  OutDataTypeStr=fixdt(1, 18, 0)  ConvertRealWorld=Stored Integer (SI)  SampleTime=1.38600138600139e-08  SaturateOnIntegerOverflow=off  RndMeth=Floor
  enb_counter_eq_0 : simulink/Logic and Bit Operations/Compare To Constant  relop===  const=double(0)  OutDataTypeStr=boolean
  enb_counter_eq_5 : simulink/Logic and Bit Operations/Compare To Constant  relop===  const=double(5)  OutDataTypeStr=boolean
  enb_counter_ge_32 : simulink/Logic and Bit Operations/Compare To Constant  relop=>=  const=double(32)  OutDataTypeStr=boolean
  enb_counter_le_4 : simulink/Logic and Bit Operations/Compare To Constant  relop=<=  const=double(4)  OutDataTypeStr=boolean
  enb_counter_le_5 : simulink/Logic and Bit Operations/Compare To Constant  relop=<=  const=double(5)  OutDataTypeStr=boolean
  gain : Gain  Gain="fi(0,0,1,4,\"hex\",\"1\")"  ParamDataTypeStr=fixdt(0, 1, 4)  OutDataTypeStr=fixdt(1, 18, 0)  SampleTime=1.38600138600139e-08
  t : Mux  Inputs=2
  t1 : Mux  Inputs=2
  tappedDelay : Subsystem
  tappedDelay1 : Subsystem
  out0 : Outport  OutDataTypeStr=fixdt(1, 18, 8)  PortDimensions=[6]  SampleTime=1.38600138600139e-08
  out1 : Outport  Port=2  OutDataTypeStr=fixdt(1, 18, 8)  PortDimensions=[6]  SampleTime=1.38600138600139e-08
  wires:
  tappedDelay/1(out0) -> Discrete-Time Integrator_u_sat_bypass/1(in0)
  enb_counter/1 -> enb_counter_ge_32/1, enb_counter_eq_5/1, enb_counter_eq_0/1, enb_counter_le_5/1, enb_counter_le_4/1
  Subtract1/1 -> HwModeRegister/1
  enb_counter_eq_5/1 -> buffSig_bypass/2(in1), buffSig_bypass1/2(in1)
  Gain3_const/1 -> HwModeRegister6/1
  Serializer_Subnetwork1/1(out0) -> delayMatch3/1
  enb_counter_le_5/1 -> counter/Enable
  enb_counter_le_4/1 -> tappedDelay1/Enable
  in0/1 -> Serializer_Subnetwork/1(in0)
  Serializer_Subnetwork3/1(out0) -> HwModeRegister3/1
  counter/1(out0) -> delayMatch5/1, delayMatch4/1, Serializer_Subnetwork1/2(in1), Serializer_Subnetwork/2(in1)
  HwModeRegister1/1 -> Multiply-Add/2
  buffSig_bypass/1(out0) -> t1/1
  in1/1 -> Serializer_Subnetwork1/1(in0)
  Serializer_Subnetwork/1(out0) -> tappedDelay1/1(in0), delayMatch2/1, delayMatch1/1, buffSig_bypass1/1(in0)
  t/1 -> out0/1
  in3/1 -> Serializer_Subnetwork3/1(in0)
  HwModeRegister2/1 -> Multiply-Add/3
  delayMatch5/1 -> Serializer_Subnetwork3/2(in1)
  delayMatch2/1 -> adder/1
  in2/1 -> Serializer_Subnetwork2/1(in0)
  Discrete-Time Integrator_u_sat_bypass1/1(out0) -> t/2
  delayMatch4/1 -> Serializer_Subnetwork2/2(in1)
  PipelineRegister2/1 -> Gain3_out_dtc/1
  tappedDelay1/1(out0) -> buffSig_bypass/1(in0)
  buffSig_bypass1/1(out0) -> t1/2
  Gain1_const/1 -> HwModeRegister4/1
  Serializer_Subnetwork2/1(out0) -> Equal/2, HwModeRegister5/1
  Gain3_out_dtc/1 -> delayMatch_absorbed/1, delayMatch_absorbed1/1
  Constant/1 -> Equal/1
  delayMatch3/1 -> OR/1
  HwModeRegister3/1 -> Gain1/1
  HwModeRegister4/1 -> Gain1/2
  HwModeRegister5/1 -> Gain3/1
  HwModeRegister6/1 -> Gain3/2
  HwModeRegister/1 -> Multiply-Add/1
  Equal/1 -> OR/2
  delayMatch/1 -> HwModeRegister1/1
  t1/1 -> out1/1
  Gain1/1 -> PipelineRegister1/1
  Gain3/1 -> PipelineRegister2/1
  OR/1 -> delayMatch/1
  PipelineRegister1/1 -> Gain1_out_dtc/1
  Gain1_out_dtc/1 -> Subtract1/1
  delayMatch_absorbed/1 -> Subtract1/2
  delayMatch_absorbed1/1 -> HwModeRegister2/1
  delayMatch1/1 -> Subtract/2
  Multiply-Add/1 -> PipelineRegister/1
  enb_counter_ge_32/1 -> tappedDelay/Enable
  PipelineRegister/1 -> Subtract/1
  Subtract/1 -> dtc1/1
  dtc1/1 -> gain/1
  gain/1 -> dtc/1
  dtc/1 -> adder/2
  adder/1 -> tappedDelay/1(in0), Discrete-Time Integrator_u_sat_bypass1/1(in0)
  enb_counter_eq_0/1 -> Discrete-Time Integrator_u_sat_bypass/2(in1), Discrete-Time Integrator_u_sat_bypass1/2(in1)
  Discrete-Time Integrator_u_sat_bypass/1(out0) -> t/1

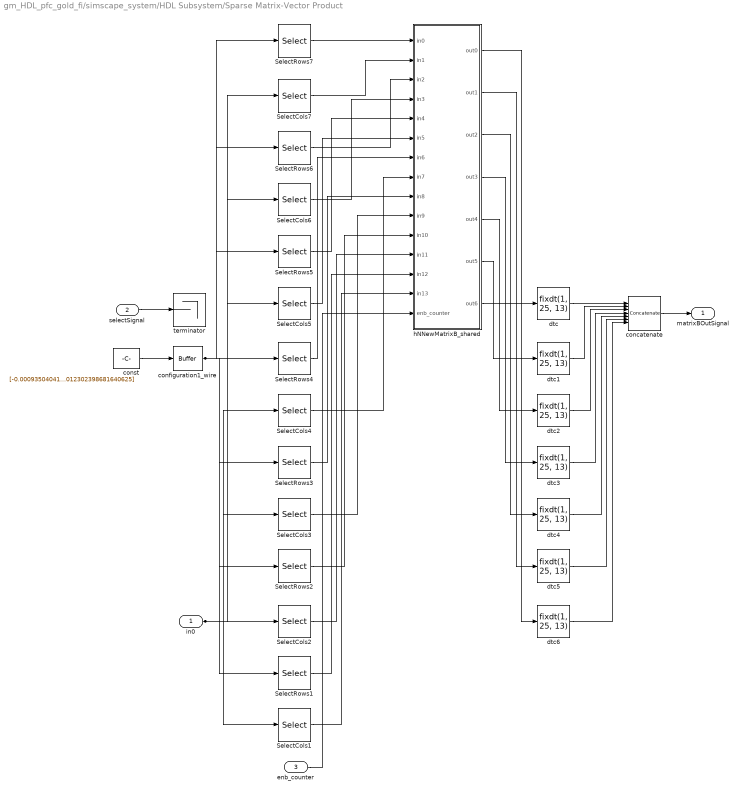
== system gm_HDL_pfc_gold_fi/simscape_system/HDL Subsystem/Sparse Matrix-Vector Product ==
  in0 : Inport  OutDataTypeStr=fixdt(1, 25, 13)  PortDimensions=[10]  SampleTime=1.38600138600139e-08
  selectSignal : Inport  Port=2  OutDataTypeStr=boolean  SampleTime=1.38600138600139e-08
  enb_counter : Inport  Port=3  OutDataTypeStr=fixdt(0, 6, 0)  SampleTime=1.38600138600139e-08
  SelectCols{1..6} (6 alike) : Selector  InputPortWidth=10  IndexOptions=Index vector (dialog)  Indices=double([2 3 4 5 6 7 8 9 10])  OutputSizes=double(1)
  SelectCols7 : Selector  InputPortWidth=10  IndexOptions=Index vector (dialog)  Indices=double([1 2 3 4 5 6 7 8 9])  OutputSizes=double(1)
  SelectRows1 : Selector  InputPortWidth=63  IndexOptions=Index vector (dialog)  Indices=double([2 9 16 23 30 37 44 51 58])  OutputSizes=double(1)
  SelectRows2 : Selector  InputPortWidth=63  IndexOptions=Index vector (dialog)  Indices=double([3 10 17 24 31 38 45 52 59])  OutputSizes=double(1)
  SelectRows3 : Selector  InputPortWidth=63  IndexOptions=Index vector (dialog)  Indices=double([4 11 18 25 32 39 46 53 60])  OutputSizes=double(1)
  SelectRows4 : Selector  InputPortWidth=63  IndexOptions=Index vector (dialog)  Indices=double([5 12 19 26 33 40 47 54 61])  OutputSizes=double(1)
  SelectRows5 : Selector  InputPortWidth=63  IndexOptions=Index vector (dialog)  Indices=double([6 13 20 27 34 41 48 55 62])  OutputSizes=double(1)
  SelectRows6 : Selector  InputPortWidth=63  IndexOptions=Index vector (dialog)  Indices=double([7 14 21 28 35 42 49 56 63])  OutputSizes=double(1)
  SelectRows7 : Selector  InputPortWidth=63  IndexOptions=Index vector (dialog)  Indices=double([1 8 15 22 29 36 43 50 57])  OutputSizes=double(1)
  concatenate : Concatenate  NumInputs=7
  configuration1_wire : hdlmdlgenlib/Buffer
  const : Constant  Value=[-0.000935040414333343505859375;0.00615119002759456634521484375;-0.003075595013797283172607421875;-0.003075595013797283172607421875;-0.003075600601732730865478515625;-0.003075600601732730865478515625;0.0061512016691267490386962890625;0.0004675202071666717529296875;-0.00615119002759456634521484375;0.003075595013797283172607421875;0.003075595013797283172607421875;0.003075600601732730865478515625;0.003075600601732730865478515625;-0.0061512016691267490386962890625;0.0004675202071666717529296875;0.003075595013797283172607421875;-0.00615119002759456634521484375;0.003075595013797283172607421875;-0.0061512016691267490386962890625;0.003075600601732730865478515625;0.003075600601732730865478515625;0.0004675202071666717529296875;0.003075595013797283172607421875;0.003075595013797283172607421875;-0.00615119002759456634521484375;0.003075600601732730865478515625;-0.0061512016691267490386962890625;0.003075600601732730865478515625;0.0004675202071666717529296875;-0.003075595013797283172607421875;0.00615119002759456634521484375;-0.003075595013797283172607421875;0.0061512016691267490386962890625;-0.003075600601732730865478515625;-0.003075600601732730865478515625;0.0004675202071666717529296875;-0.003075595013797283172607421875;-0.003075595013797283172607421875;0.00615119002759456634521484375;-0.003075600601732730865478515625;0.0061512016691267490386962890625;-0.003075600601732730865478515625;0.0004675202071666717529296875;0.0002460475079715251922607421875;-0.00012302398681640625;-0.00012302398681640625;-0.00012302398681640625;-0.00012302398681640625;0.0002460479736328125;0;-0.00012302398681640625;0.0002460475079715251922607421875;-0.00012302398681640625;0.0002460479736328125;-0.00012302398681640625;-0.00012302398681640625;0;-0.00012302398681640625;-0.00012302398681640625;0.0002460475079715251922607421875;-0.00012302398681640625;0.0002460479736328125;-0.00012302398681640625]  OutDataTypeStr=fixdt(1, 25, 31)  SampleTime=1.38600138600139e-08
  dtc{,1..6} (7 alike) : DataTypeConversion  OutDataTypeStr=fixdt(1, 25, 13)  RndMeth=Nearest  SampleTime=1.38600138600139e-08  SaturateOnIntegerOverflow=off
  hNNewMatrixB_shared : Subsystem
  terminator : Terminator
  matrixBOutSignal : Outport  OutDataTypeStr=fixdt(1, 25, 13)  PortDimensions=[7]  SampleTime=1.38600138600139e-08
  wires:
  configuration1_wire/1 -> SelectRows6/1, SelectRows5/1, SelectRows7/1, SelectRows4/1, SelectRows2/1, SelectRows3/1, SelectRows1/1
  selectSignal/1 -> terminator/1
  SelectRows7/1 -> hNNewMatrixB_shared/1(in0)
  const/1 -> configuration1_wire/1
  SelectCols7/1 -> hNNewMatrixB_shared/2(in1)
  in0/1 -> SelectCols6/1, SelectCols7/1, SelectCols3/1, SelectCols2/1, SelectCols4/1, SelectCols5/1, SelectCols1/1
  SelectRows6/1 -> hNNewMatrixB_shared/3(in2)
  SelectCols6/1 -> hNNewMatrixB_shared/4(in3)
  SelectRows5/1 -> hNNewMatrixB_shared/5(in4)
  SelectCols5/1 -> hNNewMatrixB_shared/6(in5)
  hNNewMatrixB_shared/7(out6) -> dtc/1
  SelectRows4/1 -> hNNewMatrixB_shared/7(in6)
  SelectCols4/1 -> hNNewMatrixB_shared/8(in7)
  SelectRows3/1 -> hNNewMatrixB_shared/9(in8)
  SelectCols3/1 -> hNNewMatrixB_shared/10(in9)
  hNNewMatrixB_shared/5(out4) -> dtc2/1
  SelectRows2/1 -> hNNewMatrixB_shared/11(in10)
  SelectCols2/1 -> hNNewMatrixB_shared/12(in11)
  SelectRows1/1 -> hNNewMatrixB_shared/13(in12)
  SelectCols1/1 -> hNNewMatrixB_shared/14(in13)
  enb_counter/1 -> hNNewMatrixB_shared/15(enb_counter)
  hNNewMatrixB_shared/1(out0) -> dtc6/1
  hNNewMatrixB_shared/2(out1) -> dtc5/1
  hNNewMatrixB_shared/3(out2) -> dtc4/1
  hNNewMatrixB_shared/4(out3) -> dtc3/1
  hNNewMatrixB_shared/6(out5) -> dtc1/1
  dtc/1 -> concatenate/1
  dtc1/1 -> concatenate/2
  dtc2/1 -> concatenate/3
  dtc3/1 -> concatenate/4
  dtc4/1 -> concatenate/5
  dtc5/1 -> concatenate/6
  dtc6/1 -> concatenate/7
  concatenate/1 -> matrixBOutSignal/1

== system gm_HDL_pfc_gold_fi/simscape_system/HDL Subsystem/Sparse Matrix-Vector Product1 ==
  delayOutSignal : Inport  OutDataTypeStr=fixdt(1, 25, 13)  PortDimensions=[7]  SampleTime=1.38600138600139e-08
  selectSignal : Inport  Port=2  OutDataTypeStr=boolean  SampleTime=1.38600138600139e-08
  enb_counter : Inport  Port=3  OutDataTypeStr=fixdt(0, 6, 0)  SampleTime=1.38600138600139e-08
  SelectCols{1..6} (6 alike) : Selector  InputPortWidth=7  IndexOptions=Index vector (dialog)  Indices=double([1 2 3 4 5 6])  OutputSizes=double(1)
  SelectCols7 : Selector  InputPortWidth=7  IndexOptions=Index vector (dialog)  Indices=double([1 2 3 4 5 7])  OutputSizes=double(1)
  SelectRows1 : Selector  InputPortWidth=42  IndexOptions=Index vector (dialog)  Indices=double([1 8 15 22 29 36])  OutputSizes=double(1)
  SelectRows2 : Selector  InputPortWidth=42  IndexOptions=Index vector (dialog)  Indices=double([2 9 16 23 30 37])  OutputSizes=double(1)
  SelectRows3 : Selector  InputPortWidth=42  IndexOptions=Index vector (dialog)  Indices=double([3 10 17 24 31 38])  OutputSizes=double(1)
  SelectRows4 : Selector  InputPortWidth=42  IndexOptions=Index vector (dialog)  Indices=double([4 11 18 25 32 39])  OutputSizes=double(1)
  SelectRows5 : Selector  InputPortWidth=42  IndexOptions=Index vector (dialog)  Indices=double([5 12 19 26 33 40])  OutputSizes=double(1)
  SelectRows6 : Selector  InputPortWidth=42  IndexOptions=Index vector (dialog)  Indices=double([6 13 20 27 34 41])  OutputSizes=double(1)
  SelectRows7 : Selector  InputPortWidth=42  IndexOptions=Index vector (dialog)  Indices=double([7 14 21 28 35 42])  OutputSizes=double(1)
  concatenate : Concatenate  NumInputs=7
  configuration1_wire : hdlmdlgenlib/Buffer
  const : Constant  Value=[0.559759318828582763671875;-0.27987849712371826171875;-0.27987849712371826171875;-0.279879033565521240234375;-0.279879033565521240234375;0.55975806713104248046875;0;-0.27987849712371826171875;0.559759318828582763671875;-0.27987849712371826171875;0.55975806713104248046875;-0.279879033565521240234375;-0.279879033565521240234375;0;-0.27987849712371826171875;-0.27987849712371826171875;0.559759318828582763671875;-0.279879033565521240234375;0.55975806713104248046875;-0.279879033565521240234375;0;-0.05037820339202880859375;0.100756466388702392578125;-0.05037820339202880859375;0.100757062435150146484375;-0.050378322601318359375;-0.050378322601318359375;0;-0.05037820339202880859375;-0.05037820339202880859375;0.100756466388702392578125;-0.050378322601318359375;0.100757062435150146484375;-0.050378322601318359375;0;0.100756466388702392578125;-0.05037820339202880859375;-0.05037820339202880859375;-0.050378322601318359375;-0.050378322601318359375;0.100757062435150146484375;0.999971926212310791015625]  OutDataTypeStr=fixdt(1, 25, 24)  SampleTime=1.38600138600139e-08
  dtc{,1..6} (7 alike) : DataTypeConversion  OutDataTypeStr=fixdt(1, 25, 13)  RndMeth=Nearest  SampleTime=1.38600138600139e-08  SaturateOnIntegerOverflow=off
  hNNewMatrixA_shared : Subsystem
  terminator : Terminator
  matrixAOutSignal : Outport  OutDataTypeStr=fixdt(1, 25, 13)  PortDimensions=[7]  SampleTime=1.38600138600139e-08
  wires:
  selectSignal/1 -> terminator/1
  SelectRows6/1 -> hNNewMatrixA_shared/3(in2)
  configuration1_wire/1 -> SelectRows7/1, SelectRows4/1, SelectRows5/1, SelectRows3/1, SelectRows2/1, SelectRows6/1, SelectRows1/1
  const/1 -> configuration1_wire/1
  delayOutSignal/1 -> SelectCols5/1, SelectCols3/1, SelectCols2/1, SelectCols4/1, SelectCols6/1, SelectCols1/1, SelectCols7/1
  SelectRows7/1 -> hNNewMatrixA_shared/1(in0)
  SelectCols7/1 -> hNNewMatrixA_shared/2(in1)
  SelectCols6/1 -> hNNewMatrixA_shared/4(in3)
  SelectRows5/1 -> hNNewMatrixA_shared/5(in4)
  enb_counter/1 -> hNNewMatrixA_shared/15(enb_counter)
  SelectCols5/1 -> hNNewMatrixA_shared/6(in5)
  SelectRows4/1 -> hNNewMatrixA_shared/7(in6)
  SelectCols4/1 -> hNNewMatrixA_shared/8(in7)
  SelectRows3/1 -> hNNewMatrixA_shared/9(in8)
  SelectCols3/1 -> hNNewMatrixA_shared/10(in9)
  hNNewMatrixA_shared/6(out5) -> dtc1/1
  SelectRows2/1 -> hNNewMatrixA_shared/11(in10)
  SelectCols2/1 -> hNNewMatrixA_shared/12(in11)
  SelectRows1/1 -> hNNewMatrixA_shared/13(in12)
  SelectCols1/1 -> hNNewMatrixA_shared/14(in13)
  hNNewMatrixA_shared/1(out0) -> dtc6/1
  hNNewMatrixA_shared/2(out1) -> dtc5/1
  hNNewMatrixA_shared/3(out2) -> dtc4/1
  hNNewMatrixA_shared/4(out3) -> dtc3/1
  hNNewMatrixA_shared/5(out4) -> dtc2/1
  hNNewMatrixA_shared/7(out6) -> dtc/1
  dtc/1 -> concatenate/1
  dtc1/1 -> concatenate/2
  dtc2/1 -> concatenate/3
  dtc3/1 -> concatenate/4
  dtc4/1 -> concatenate/5
  dtc5/1 -> concatenate/6
  dtc6/1 -> concatenate/7
  concatenate/1 -> matrixAOutSignal/1
